simulink model "lab7_sl"  (R2021b)
settings: Solver=ode45  StartTime=0.0  StopTime=15.0  MaxStep=2^-5  RelTol=1e-3
settings Model: Creator=JaSzw  LastModifiedBy=JaSzw

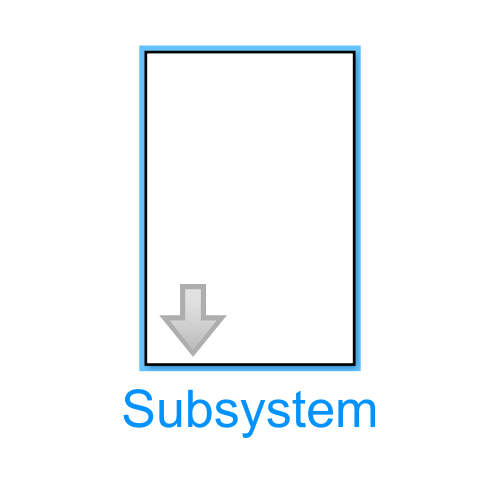
[thumbnail: Simulink's stored preview of the top-level diagram]
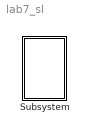
== system lab7_sl ==
  Subsystem : Subsystem  mask{th1=80, th2=150, th1p=0, th2p=0, g=9.81, k1=2, k2=1, m1=1, m2=2, l1=1, l2=2}

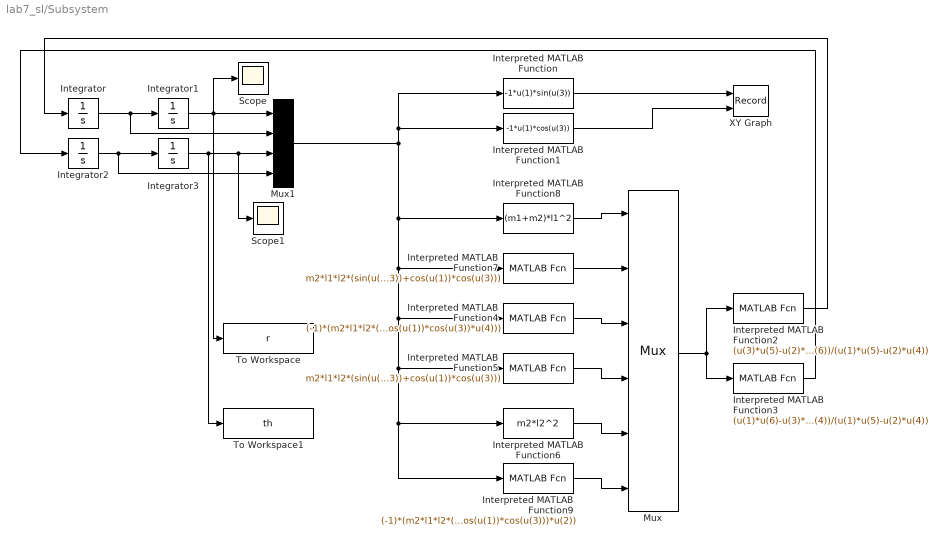
== system lab7_sl/Subsystem ==
  Integrator : Integrator  InitialCondition=th1p*pi/180
  Integrator1 : Integrator  InitialCondition=th1*pi/180
  Integrator2 : Integrator  InitialCondition=th2p*pi/180
  Integrator3 : Integrator  InitialCondition=th2*pi/180
  Interpreted MATLAB Function : MATLABFcn  MATLABFcn=-1*u(1)*sin(u(3))  OutputDimensions=1
  Interpreted MATLAB Function1 : MATLABFcn  MATLABFcn=-1*u(1)*cos(u(3))  OutputDimensions=1
  Interpreted MATLAB Function2 : MATLABFcn  MATLABFcn=(u(3)*u(5)-u(2)*u(6))/(u(1)*u(5)-u(2)*u(4))  OutputDimensions=1
  Interpreted MATLAB Function3 : MATLABFcn  MATLABFcn=(u(1)*u(6)-u(3)*u(4))/(u(1)*u(5)-u(2)*u(4))  OutputDimensions=1
  Interpreted MATLAB Function4 : MATLABFcn  MATLABFcn=(-1)*(m2*l1*l2*(sin(u(1))*cos(u(3))-cos(u(1))*sin(u(3)))*u(4)^2+(m1+m2)*g*l1*sin(u(1))+k1*l1^2*u(2)+k2*l1*l2*(sin(u(1))*sin(u(3))+cos(u(1))*cos(u(3))*u(4)))
  Interpreted MATLAB Function5 : MATLABFcn  MATLABFcn=m2*l1*l2*(sin(u(1))*sin(u(3))+cos(u(1))*cos(u(3)))  OutputDimensions=1
  Interpreted MATLAB Function6 : MATLABFcn  MATLABFcn=m2*l2^2  OutputDimensions=1
  Interpreted MATLAB Function7 : MATLABFcn  MATLABFcn=m2*l1*l2*(sin(u(1))*sin(u(3))+cos(u(1))*cos(u(3)))
  Interpreted MATLAB Function8 : MATLABFcn  MATLABFcn=(m1+m2)*l1^2
  Interpreted MATLAB Function9 : MATLABFcn  MATLABFcn=(-1)*(m2*l1*l2*(cos(u(1))*sin(u(3))-sin(u(1))*cos(u(3)))*u(2)^2+m2*g*l2*sin(u(3))+k2*l2^2*u(4)+k2*l1*l2*(sin(u(1))*sin(u(3))+cos(u(1))*cos(u(3)))*u(2))  OutputDimensions=1
  Mux : Mux  Inputs=6
  Mux1 : Mux
  Scope : Scope
  Scope1 : Scope
  To Workspace : ToWorkspace  VariableName=r  SampleTime=-1
  To Workspace1 : ToWorkspace  VariableName=th  SampleTime=-1
  XY Graph : Record  FileSettingsInternal="{\"entries\":[{\"content\":{\"excelSettings\":{\"content\":{},\"type\":\"Streamout.ExcelSettings\"}},\"type\":\"Streamout.FileSettingStorage\",\"uuid\":\"1b55d0f7-7fa7-40da-9738-d9564284a9c0\"}],\"packageUris\":[\"http://schema.mathworks.com/mf0/streamout_blocks/R2020a\"],\"version\":\"1.0\"}"  Layout=[1 1]  SignalsInternal="{\"entries\":[{\"content\":{\"signals\":[{\"content\":{\"blockPath\":[\"lab6_sl/Subsystem/XY Graph\"],\"channel\":[],\"dimensions\":[1],\"domain\":\"lab6_sl/Subsystem/XY Graph\",\"lineColor\":\"#a2142f\",\"plots\":[1],\"port\":1,\"sid\":[\"\"],\"signalID\":276,\"signalName\":\"Interpreted MATLAB\\nFunction\"},\"type\":\"RecordBlkView.Signal\",\"uuid\":\"2edacaca-8710-4cf9-ba7c-45163d0e6a09\"},{\"content\":{\"blockPath\":[\"lab6_sl/Subsystem/XY Graph\"],\"channel\":[],\"dimensions\":[1],\"domain\":\"lab6_sl/Subsystem/XY Graph\",\"lineColor\":\"#139fff\",\"plots\":[1],\"port\":2,\"sid\":[\"\"],\"signalID\":280,\"signalName\":\"Interpreted MATLAB\\nFunction1\"},\"type\":\"RecordBlkView.Signal\",\"uuid\":\"0cdc2c3d-5eb4-4860-ac41-0e8470cb520d\"}]},\"type\":\"RecordBlkView.InputSignals\",\"uuid\":\"1d4a5cbc-2f7c-4c39-b51e-1d5b26da8369\"}],\"packageUris\":[\"http://schema.mathworks.com/mf0/streamout_blocks/R2020a\"],\"version\":\"1.0\"}"  VisualizationBindings="{\"xyplotplugin\":{\"info\":[{\"series\":[{\"bindingParametersList\":[{\"parameter\":\"X-Axis\",\"signalID\":276,\"signalName\":\"Interpreted MATLAB\\nFunction\"},{\"parameter\":\"Y-Axis\",\"signalID\":280,\"signalName\":\"Interpreted MATLAB\\nFunction1\"}],\"seriesID\":24355}],\"subplotID\":1}]}}"  CompatibilityTag=XY
  wires:
  Integrator3/1 -> To Workspace1/1, Scope1/1, Mux1/3
  Mux/1 -> Interpreted MATLAB Function3/1, Interpreted MATLAB Function2/1
  Integrator2/1 -> Mux1/4, Integrator3/1
  Mux1/1 -> Interpreted MATLAB Function/1, Interpreted MATLAB Function1/1, Interpreted MATLAB Function9/1, Interpreted MATLAB Function6/1, Interpreted MATLAB Function5/1, Interpreted MATLAB Function4/1, Interpreted MATLAB Function7/1, Interpreted MATLAB Function8/1
  Interpreted MATLAB Function7/1 -> Mux/2
  Interpreted MATLAB Function1/1 -> XY Graph/2
  Integrator1/1 -> To Workspace/1, Mux1/1, Scope/1
  Interpreted MATLAB Function2/1 -> Integrator/1
  Interpreted MATLAB Function/1 -> XY Graph/1
  Integrator/1 -> Mux1/2, Integrator1/1
  Interpreted MATLAB Function3/1 -> Integrator2/1
  Interpreted MATLAB Function8/1 -> Mux/1
  Interpreted MATLAB Function9/1 -> Mux/6
  Interpreted MATLAB Function6/1 -> Mux/5
  Interpreted MATLAB Function4/1 -> Mux/3
  Interpreted MATLAB Function5/1 -> Mux/4
